simulink model "SFB_L"  (Simulink 6.6)
settings: Solver=ode5  StartTime=0.0  StopTime=50  FixedStep=0.001  RelTol=1e-3
InitFcn:
  | linmod1
undefined symbols (not defined in the file or in its folder): A, B, C, D, K
settings Model: Creator=AF1  LastModifiedBy=AF1
settings DataIOCC: SignalLoggingName=sigsOut
settings OptimizationCC: BooleanDataType=off
settings DebuggingCC: SignalResolutionControl=TryResolveAllWithWarning  SolverPrmCheckMsg=none  MultiTaskDSMMsg=warning  MultiTaskCondExecSysMsg=none  StrictBusMsg=None
settings HardwareCC: TargetUnknown=on
settings RTWCC: IncludeERTFirstTime=on

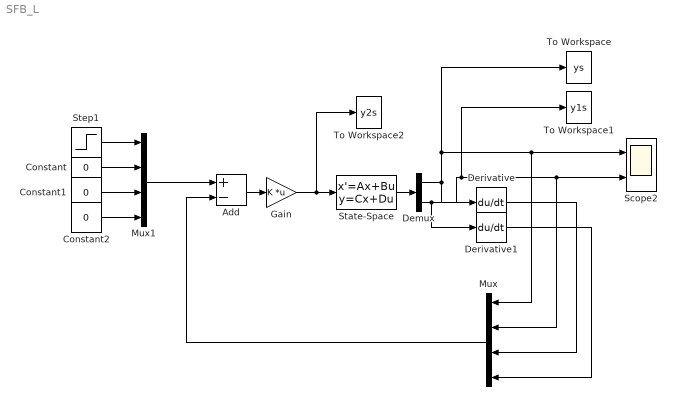
== system SFB_L ==
  Add : Sum  Inputs=+-  OutScaling=2^-10
  Constant : Constant  Value=0
  Constant1 : Constant  Value=0
  Constant2 : Constant  Value=0
  Demux : Demux  Outputs=2
  Derivative : Derivative
  Derivative1 : Derivative
  Gain : Gain  Gain=K  Multiplication=Matrix(K*u)
  Mux : Mux  Orientation=left
  Mux1 : Mux
  Scope2 : Scope  NumInputPorts=2
      settings: TimeRange=50  YMin=-0.05~-0.06  YMax=0.2~0.01000000000000001  SaveName=ScopeData2
  State-Space : StateSpace  A=A  B=B  C=C  D=D
  Step1 : Step  Time=20  After=0.2  SampleTime=0
  To Workspace : ToWorkspace  VariableName=ys  SampleTime=-1  SaveFormat=Structure With Time
  To Workspace1 : ToWorkspace  VariableName=y1s  SampleTime=-1  SaveFormat=Structure With Time
  To Workspace2 : ToWorkspace  VariableName=y2s  SampleTime=-1  SaveFormat=Structure With Time
  wires:
  Add/1 -> Gain/1
  Demux/1 -> Derivative/1, Scope2/1, Mux/1, To Workspace/1
  Demux/2 -> Derivative1/1, Scope2/2, Mux/2, To Workspace1/1
  Step1/1 -> Mux1/1
  Mux1/1 -> Add/1
  Constant/1 -> Mux1/2
  Constant1/1 -> Mux1/3
  Constant2/1 -> Mux1/4
  Gain/1 -> State-Space/1, To Workspace2/1
  State-Space/1 -> Demux/1
  Derivative/1 -> Mux/3
  Derivative1/1 -> Mux/4
  Mux/1 -> Add/2
